simulink model "Lateral_Beam_Guidance_System_Block_Diagram"  (R2025b)
settings: Solver=ode4  StartTime=0.0  StopTime=250  FixedStep=stepsize  RelTol=1e-3
values from neighbouring files (symbols this model uses):
  B_SM = 0.7    [ILS_Lateral_Beam_Guidance_System_JoshuaYandoc.m]
  g = 9.81    [ILS_Lateral_Beam_Guidance_System_JoshuaYandoc.m]
  G_c = 25.5    [ILS_Lateral_Beam_Guidance_System_JoshuaYandoc.m]
  J_M = 0.006    [ILS_Lateral_Beam_Guidance_System_JoshuaYandoc.m]
  K_A = 1.2    [ILS_Lateral_Beam_Guidance_System_JoshuaYandoc.m]
  K_D = 0.9    [ILS_Lateral_Beam_Guidance_System_JoshuaYandoc.m]
  K_E = 0.9    [ILS_Lateral_Beam_Guidance_System_JoshuaYandoc.m]
  K_P = 52.5    [ILS_Lateral_Beam_Guidance_System_JoshuaYandoc.m]
  K_R = 1.2    [ILS_Lateral_Beam_Guidance_System_JoshuaYandoc.m]
  K_T = 1.7    [ILS_Lateral_Beam_Guidance_System_JoshuaYandoc.m]
  K_V = 1.3    [ILS_Lateral_Beam_Guidance_System_JoshuaYandoc.m]
  L_A = 0.2    [ILS_Lateral_Beam_Guidance_System_JoshuaYandoc.m]
  phi_0 = deg2rad(0)    [ILS_Lateral_Beam_Guidance_System_JoshuaYandoc.m]
  psi_0 = deg2rad(-20)    [ILS_Lateral_Beam_Guidance_System_JoshuaYandoc.m]
  R = R_0    (= 6000)    [ILS_Lateral_Beam_Guidance_System_JoshuaYandoc.m]
  R_A = 10    [ILS_Lateral_Beam_Guidance_System_JoshuaYandoc.m]
  T_A = 2.0    (= 2)    [ILS_Lateral_Beam_Guidance_System_JoshuaYandoc.m]
  V_T = 60    [ILS_Lateral_Beam_Guidance_System_JoshuaYandoc.m]
libraries: simulink_extras x5
settings Model: Creator=jyand  LastModifiedBy=Joshua
settings DataIOCC: SaveFormat=Array  SaveOutput=off  SignalLogging=off

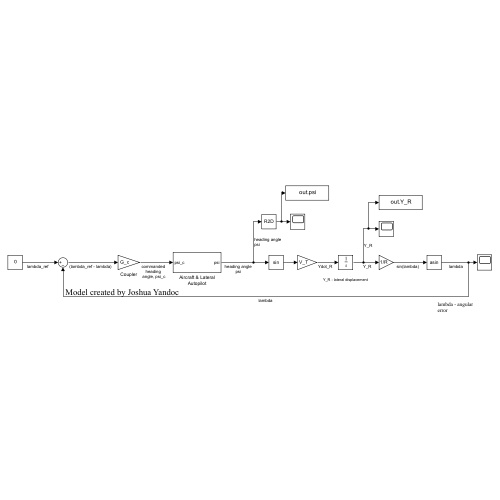
[thumbnail: Simulink's stored preview of the top-level diagram]
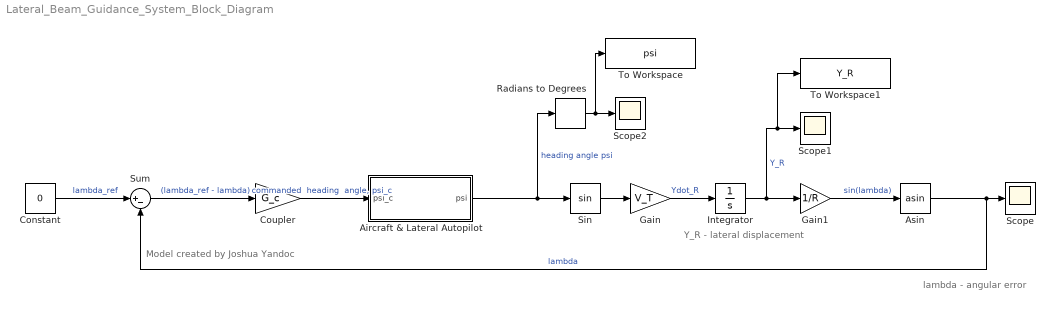
== system Lateral_Beam_Guidance_System_Block_Diagram ==
  note: Model created by Joshua Yandoc
  note: Y_R - lateral displacement
  note: lambda - angular
      | error
  Aircraft & Lateral Autopilot : Subsystem
  Asin : Trigonometry  Operator=asin
  Constant : Constant  Value=0
  Coupler : Gain  Gain=G_c
  Gain : Gain  Gain=V_T
  Gain1 : Gain  Gain=1/R
  Integrator : Integrator  InitialCondition=150
  Radians to Degrees : simulink_extras/Transformations/Radians to Degrees
  Scope : Scope
      settings: ActiveDisplayYMinimum=-0.02171  ActiveDisplayYMaximum=0.03019
  Scope1 : Scope
      settings: ActiveDisplayYMinimum=-1  ActiveDisplayYMaximum=1  DataLoggingVariableName=ScopeData4
  Scope2 : Scope
      settings: ActiveDisplayYMinimum=-1  ActiveDisplayYMaximum=1  DataLoggingVariableName=ScopeData5
  Sin : Trigonometry
  Sum : Sum  Inputs=|+-
  To Workspace : ToWorkspace  VariableName=psi  SampleTime=-1
  To Workspace1 : ToWorkspace  VariableName=Y_R  SampleTime=-1
  wires:
  Sum/1 -> Coupler/1  "(lambda_ref - lambda)"
  Constant/1 -> Sum/1  "lambda_ref"
  Asin/1 -> Sum/2, Scope/1  "lambda"
  Coupler/1 -> Aircraft & Lateral Autopilot/1(psi_c)  "commanded  heading  angle, psi_c"
  Aircraft & Lateral Autopilot/1(psi) -> Sin/1, Radians to Degrees/1  "heading angle psi"
  Sin/1 -> Gain/1
  Gain/1 -> Integrator/1  "Ydot_R"
  Integrator/1 -> To Workspace1/1, Scope1/1, Gain1/1  "Y_R"
  Gain1/1 -> Asin/1  "sin(lambda)"
  Radians to Degrees/1 -> To Workspace/1, Scope2/1

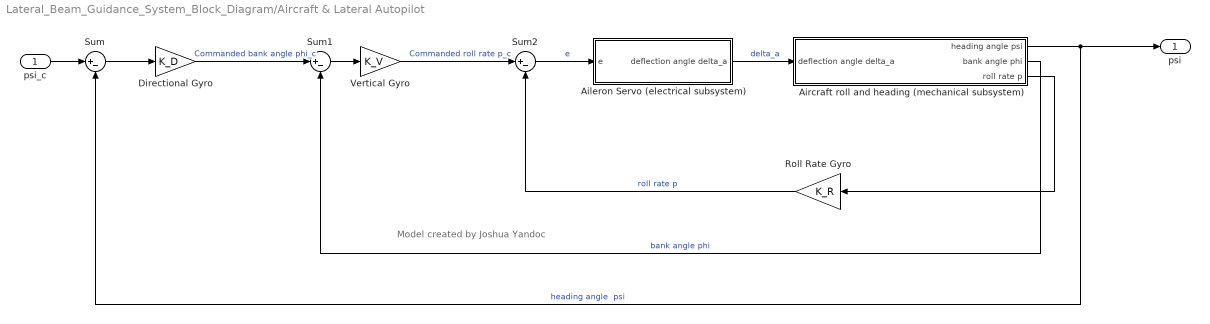
== system Lateral_Beam_Guidance_System_Block_Diagram/Aircraft & Lateral Autopilot ==
  note: Model created by Joshua Yandoc
  psi_c : Inport
  "Aileron Servo (electrical subsystem) " : Subsystem
  Aircraft roll and heading (mechanical subsystem) : Subsystem
  Directional Gyro : Gain  Gain=K_D
  Roll Rate Gyro : Gain  Gain=K_R
  Sum : Sum  Inputs=|+-
  Sum1 : Sum  Inputs=|+-
  Sum2 : Sum  Inputs=|+-
  Vertical Gyro : Gain  Gain=K_V
  psi : Outport
  wires:
  psi_c/1 -> Sum/1
  Sum/1 -> Directional Gyro/1
  Directional Gyro/1 -> Sum1/1  "Commanded bank angle phi_c"
  Sum1/1 -> Vertical Gyro/1
  Vertical Gyro/1 -> Sum2/1  "Commanded roll rate p_c"
  Sum2/1 -> "Aileron Servo (electrical subsystem) "/1(e)  "e"
  "Aileron Servo (electrical subsystem) "/1(deflection angle delta_a) -> Aircraft roll and heading (mechanical subsystem)/1(deflection angle delta_a)  "delta_a"
  Aircraft roll and heading (mechanical subsystem)/1(heading angle psi) -> Sum/2, psi/1  "heading angle  psi"
  Aircraft roll and heading (mechanical subsystem)/2(bank angle phi) -> Sum1/2  "bank angle phi"
  Aircraft roll and heading (mechanical subsystem)/3(roll rate p) -> Roll Rate Gyro/1
  Roll Rate Gyro/1 -> Sum2/2  "roll rate p"

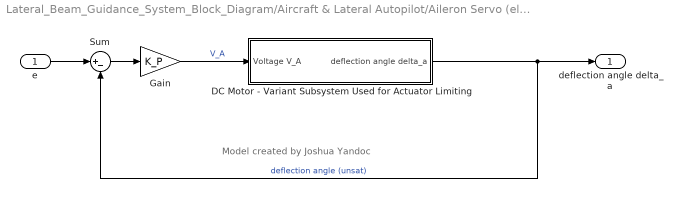
== system Lateral_Beam_Guidance_System_Block_Diagram/Aircraft & Lateral Autopilot/Aileron Servo (electrical subsystem)  ==
  note: Model created by Joshua Yandoc
  e : Inport
  DC Motor - Variant Subsystem Used for Actuator Limiting : Subsystem
  Gain : Gain  Gain=K_P
  Sum : Sum  Inputs=|+-
  deflection angle delta_a : Outport
  wires:
  e/1 -> Sum/1
  Sum/1 -> Gain/1
  Gain/1 -> DC Motor - Variant Subsystem Used for Actuator Limiting/1(Voltage V_A)  "V_A"
  DC Motor - Variant Subsystem Used for Actuator Limiting/1(deflection angle delta_a) -> deflection angle delta_a/1, Sum/2  "deflection angle (unsat)"

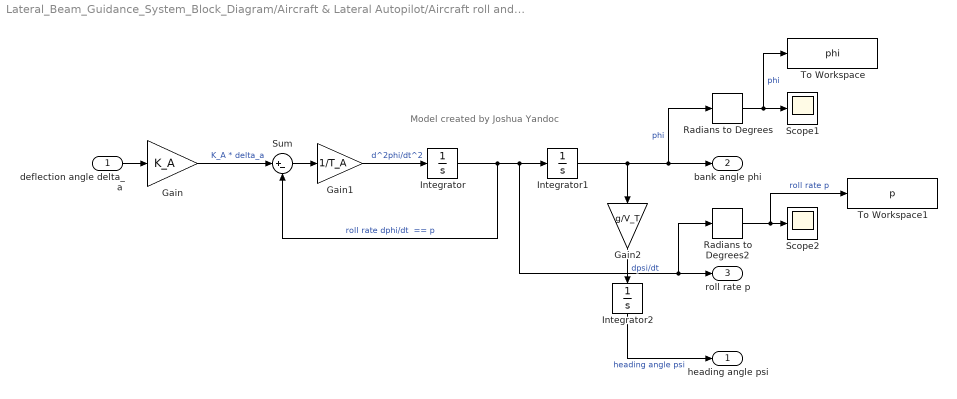
== system Lateral_Beam_Guidance_System_Block_Diagram/Aircraft & Lateral Autopilot/Aircraft roll and heading (mechanical subsystem) ==
  note: Model created by Joshua Yandoc
  deflection angle delta_a : Inport
  Gain : Gain  Gain=K_A
  Gain1 : Gain  Gain=1/T_A
  Gain2 : Gain  Gain=g/V_T
  Integrator : Integrator
  Integrator1 : Integrator  InitialCondition=phi_0
  Integrator2 : Integrator  InitialCondition=psi_0
  Radians to Degrees : simulink_extras/Transformations/Radians to Degrees
  Radians to Degrees2 : simulink_extras/Transformations/Radians to Degrees
  Scope1 : Scope
      settings: ActiveDisplayYMinimum=-46.5809  ActiveDisplayYMaximum=58.67229  DataLoggingVariableName=ScopeData2
  Scope2 : Scope
      settings: ActiveDisplayYMinimum=-18.73362  ActiveDisplayYMaximum=19.26047  DataLoggingVariableName=ScopeData3
  Sum : Sum  Inputs=|+-
  To Workspace : ToWorkspace  VariableName=phi  SampleTime=-1
  To Workspace1 : ToWorkspace  VariableName=p  SampleTime=-1
  heading angle psi : Outport
  bank angle phi : Outport  Port=2
  roll rate p : Outport  Port=3
  wires:
  deflection angle delta_a/1 -> Gain/1
  Gain/1 -> Sum/1  "K_A * delta_a"
  Sum/1 -> Gain1/1
  Gain1/1 -> Integrator/1  "d^2phi/dt^2"
  Integrator/1 -> Radians to Degrees2/1, roll rate p/1, Integrator1/1, Sum/2  "roll rate dphi/dt  == p"
  Integrator1/1 -> Radians to Degrees/1, bank angle phi/1, Gain2/1  "phi"
  Gain2/1 -> Integrator2/1  "dpsi/dt"
  Integrator2/1 -> heading angle psi/1  "heading angle psi"
  Radians to Degrees/1 -> To Workspace/1, Scope1/1  "phi"
  Radians to Degrees2/1 -> To Workspace1/1, Scope2/1  "roll rate p"

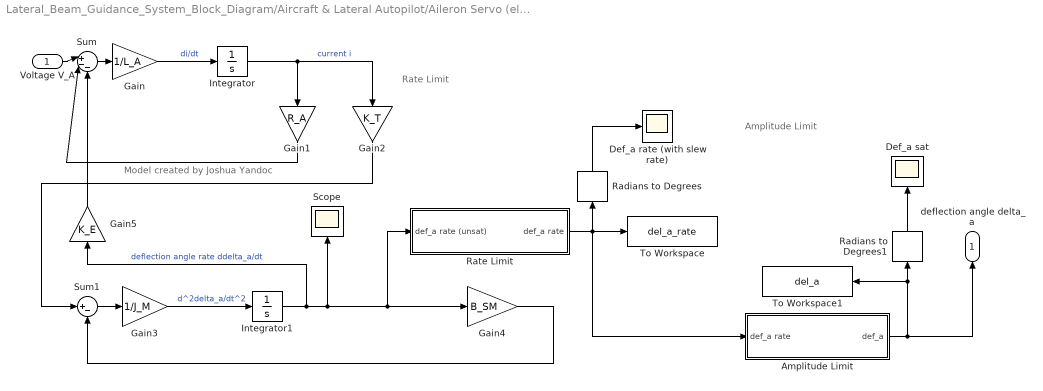
== system Lateral_Beam_Guidance_System_Block_Diagram/Aircraft & Lateral Autopilot/Aileron Servo (electrical subsystem) /DC Motor - Variant Subsystem Used for Actuator Limiting ==
  note: Amplitude Limit
  note: Rate Limit
  note: Model created by Joshua Yandoc
  Voltage V_A : Inport
  Amplitude Limit : Subsystem  Variant=on
  Def_a sat : Scope
      settings: ActiveDisplayYMinimum=-1  ActiveDisplayYMaximum=1  DataLoggingVariableName=ScopeData7
  Def_a rate (with slew rate) : Scope
      settings: ActiveDisplayYMinimum=-186.1133897539878  ActiveDisplayYMaximum=40.823593205519693  DataLoggingVariableName=ScopeData6
  Gain : Gain  Gain=1/L_A
  Gain1 : Gain  Gain=R_A
  Gain2 : Gain  Gain=K_T
  Gain3 : Gain  Gain=1/J_M
  Gain4 : Gain  Gain=B_SM
  Gain5 : Gain  Gain=K_E
  Integrator : Integrator
  Integrator1 : Integrator
  Radians to Degrees : simulink_extras/Transformations/Radians to Degrees
  Radians to Degrees1 : simulink_extras/Transformations/Radians to Degrees
  Rate Limit : Subsystem  Variant=on
  Scope : Scope
      settings: ActiveDisplayYMinimum=-1  ActiveDisplayYMaximum=1  DataLoggingVariableName=ScopeData8
  Sum : Sum  Inputs=|+--
  Sum1 : Sum  Inputs=|+-
  To Workspace : ToWorkspace  VariableName=del_a_rate  SampleTime=-1
  To Workspace1 : ToWorkspace  VariableName=del_a  SampleTime=-1
  deflection angle delta_a : Outport
  wires:
  Voltage V_A/1 -> Sum/1
  Sum/1 -> Gain/1
  Gain/1 -> Integrator/1  "di/dt"
  Integrator/1 -> Gain2/1, Gain1/1  "current i"
  Gain1/1 -> Sum/2
  Gain2/1 -> Sum1/1
  Sum1/1 -> Gain3/1
  Gain3/1 -> Integrator1/1  "d^2delta_a/dt^2"
  Integrator1/1 -> Rate Limit/1(def_a rate (unsat)), Gain4/1, Scope/1, Gain5/1  "deflection angle rate ddelta_a/dt"
  Gain4/1 -> Sum1/2
  Gain5/1 -> Sum/3
  Rate Limit/1(def_a rate) -> Amplitude Limit/1(def_a rate), To Workspace/1, Radians to Degrees/1
  Radians to Degrees/1 -> Def_a rate (with slew rate)/1
  Amplitude Limit/1(def_a) -> To Workspace1/1, Radians to Degrees1/1, deflection angle delta_a/1
  Radians to Degrees1/1 -> Def_a sat/1

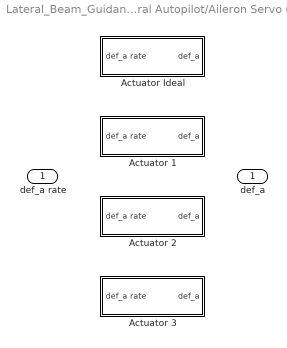
== system Lateral_Beam_Guidance_System_Block_Diagram/Aircraft & Lateral Autopilot/Aileron Servo (electrical subsystem) /DC Motor - Variant Subsystem Used for Actuator Limiting/Amplitude Limit ==
  def_a rate : Inport
  Actuator 1 : Subsystem  VariantControl=USE_ACTUATOR == 1
  Actuator 2 : Subsystem  VariantControl=USE_ACTUATOR == 2
  Actuator 3 : Subsystem  VariantControl=USE_ACTUATOR == 3
  Actuator Ideal : Subsystem  VariantControl=USE_ACTUATOR == -1
  def_a : Outport

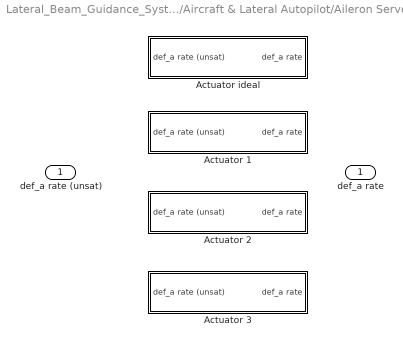
== system Lateral_Beam_Guidance_System_Block_Diagram/Aircraft & Lateral Autopilot/Aileron Servo (electrical subsystem) /DC Motor - Variant Subsystem Used for Actuator Limiting/Rate Limit ==
  def_a rate (unsat) : Inport
  Actuator 1 : Subsystem  VariantControl=USE_ACTUATOR == 1
  Actuator 2 : Subsystem  VariantControl=USE_ACTUATOR == 2
  Actuator 3 : Subsystem  VariantControl=USE_ACTUATOR == 3
  Actuator ideal : Subsystem  VariantControl=USE_ACTUATOR == -1
  def_a rate : Outport

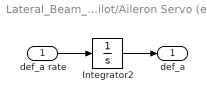
== system Lateral_Beam_Guidance_System_Block_Diagram/Aircraft & Lateral Autopilot/Aileron Servo (electrical subsystem) /DC Motor - Variant Subsystem Used for Actuator Limiting/Amplitude Limit/Actuator 1 ==
  def_a rate : Inport
  Integrator2 : Integrator  LimitOutput=on  UpperSaturationLimit=10 * (pi/180)  LowerSaturationLimit=-10 * (pi/180)
  def_a : Outport
  wires:
  Integrator2/1 -> def_a/1
  def_a rate/1 -> Integrator2/1

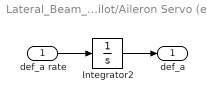
== system Lateral_Beam_Guidance_System_Block_Diagram/Aircraft & Lateral Autopilot/Aileron Servo (electrical subsystem) /DC Motor - Variant Subsystem Used for Actuator Limiting/Amplitude Limit/Actuator 2 ==
  def_a rate : Inport
  Integrator2 : Integrator  LimitOutput=on  UpperSaturationLimit=15 * (pi/180)  LowerSaturationLimit=-15 * (pi/180)
  def_a : Outport
  wires:
  Integrator2/1 -> def_a/1
  def_a rate/1 -> Integrator2/1

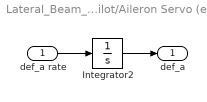
== system Lateral_Beam_Guidance_System_Block_Diagram/Aircraft & Lateral Autopilot/Aileron Servo (electrical subsystem) /DC Motor - Variant Subsystem Used for Actuator Limiting/Amplitude Limit/Actuator 3 ==
  def_a rate : Inport
  Integrator2 : Integrator  LimitOutput=on  UpperSaturationLimit=20 * (pi/180)  LowerSaturationLimit=-20 * (pi/180)
  def_a : Outport
  wires:
  Integrator2/1 -> def_a/1
  def_a rate/1 -> Integrator2/1

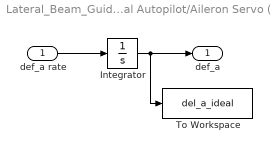
== system Lateral_Beam_Guidance_System_Block_Diagram/Aircraft & Lateral Autopilot/Aileron Servo (electrical subsystem) /DC Motor - Variant Subsystem Used for Actuator Limiting/Amplitude Limit/Actuator Ideal ==
  def_a rate : Inport
  Integrator : Integrator
  To Workspace : ToWorkspace  VariableName=del_a_ideal  SampleTime=-1
  def_a : Outport
  wires:
  def_a rate/1 -> Integrator/1
  Integrator/1 -> To Workspace/1, def_a/1

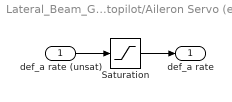
== system Lateral_Beam_Guidance_System_Block_Diagram/Aircraft & Lateral Autopilot/Aileron Servo (electrical subsystem) /DC Motor - Variant Subsystem Used for Actuator Limiting/Rate Limit/Actuator 1 ==
  def_a rate (unsat) : Inport
  Saturation : Saturate  UpperLimit=5 * (pi/180)  LowerLimit=-5 * (pi/180)
  def_a rate : Outport
  wires:
  def_a rate (unsat)/1 -> Saturation/1
  Saturation/1 -> def_a rate/1

== system Lateral_Beam_Guidance_System_Block_Diagram/Aircraft & Lateral Autopilot/Aileron Servo (electrical subsystem) /DC Motor - Variant Subsystem Used for Actuator Limiting/Rate Limit/Actuator 2 ==
  def_a rate (unsat) : Inport
  Saturation : Saturate  UpperLimit=7.5 * (pi/180)  LowerLimit=-7.5 * (pi/180)
  def_a rate : Outport
  wires:
  def_a rate (unsat)/1 -> Saturation/1
  Saturation/1 -> def_a rate/1

== system Lateral_Beam_Guidance_System_Block_Diagram/Aircraft & Lateral Autopilot/Aileron Servo (electrical subsystem) /DC Motor - Variant Subsystem Used for Actuator Limiting/Rate Limit/Actuator 3 ==
  def_a rate (unsat) : Inport
  Saturation : Saturate  UpperLimit=10 * (pi/180)  LowerLimit=-10 * (pi/180)
  def_a rate : Outport
  wires:
  def_a rate (unsat)/1 -> Saturation/1
  Saturation/1 -> def_a rate/1

== system Lateral_Beam_Guidance_System_Block_Diagram/Aircraft & Lateral Autopilot/Aileron Servo (electrical subsystem) /DC Motor - Variant Subsystem Used for Actuator Limiting/Rate Limit/Actuator ideal ==
  def_a rate (unsat) : Inport
  def_a rate : Outport
  wires:
  def_a rate (unsat)/1 -> def_a rate/1
